simulink model "LevelControl_2025b"  (R2025b)
settings: Solver=FixedStepAuto  StartTime=0.0  StopTime=inf  RelTol=1e-3  EnableMultiTasking=on
libraries: dspstat3 x2, slpidlib x1, arduinolib x1, arduinosensorlib x1
settings Model: ExtModeTrigDuration=2  Creator=Arnt Inge Bøe  LastModifiedBy=Arnt Inge Bøe
settings SolverCC: AutoInsertRateTranBlk=on
settings DataIOCC: ReturnWorkspaceOutputs=off
settings OptimizationCC: EnhancedBackFolding=on  PassReuseOutputArgsAs=Individual arguments  ZeroExternalMemoryAtStartup=off  ZeroInternalMemoryAtStartup=off  MaxStackSize=64  OptimizeBlockOrder=speed  DifferentSizesBufferReuse=on  EfficientTunableParamExpr=on
settings DebuggingCC: ParameterTunabilityLossMsg=error
settings HardwareCC: ProdBitPerPointer=32.0  ProdBitPerSizeT=32.0  ProdBitPerPtrDiffT=32.0  ProdLargestAtomicInteger=Long  ProdLargestAtomicFloat=Double  ProdWordSize=32.0  ProdHWDeviceType=ARM Compatible->ARM Cortex
settings SFSimCC: MATLABDynamicMemAlloc=off
settings RTWCC: SystemTargetFile=ert.tlc  HardwareBoard=Arduino Uno R4 WiFi  TemplateMakefile=ert_default_tmf  Toolchain=Arduino ARM M4  BuildConfiguration=Faster Runs  Description=Embedded Coder
settings CodeAppCC: ForceParamTrailComments=on  IgnoreCustomStorageClasses=off  OperatorAnnotations=on  SimulinkDataObjDesc=on  SFDataObjDesc=on  InsertBlockDesc=on
settings ERTTargetCC: ExtModeTransport=3.0  ExtModeStaticAlloc=on  ExtModeAutomaticAllocSize=off  ExtModeStaticAllocSize=8192.0  ExtModeMexFile=ext_xcp  ExtModeIntrfLevel=Level2 - Open  InlinedParameterPlacement=Hierarchical  SupportContinuousTime=on  SupportVariableSizeSignals=on

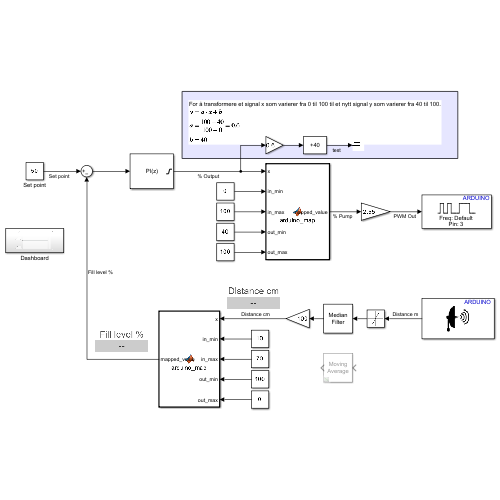
[thumbnail: Simulink's stored preview of the top-level diagram]
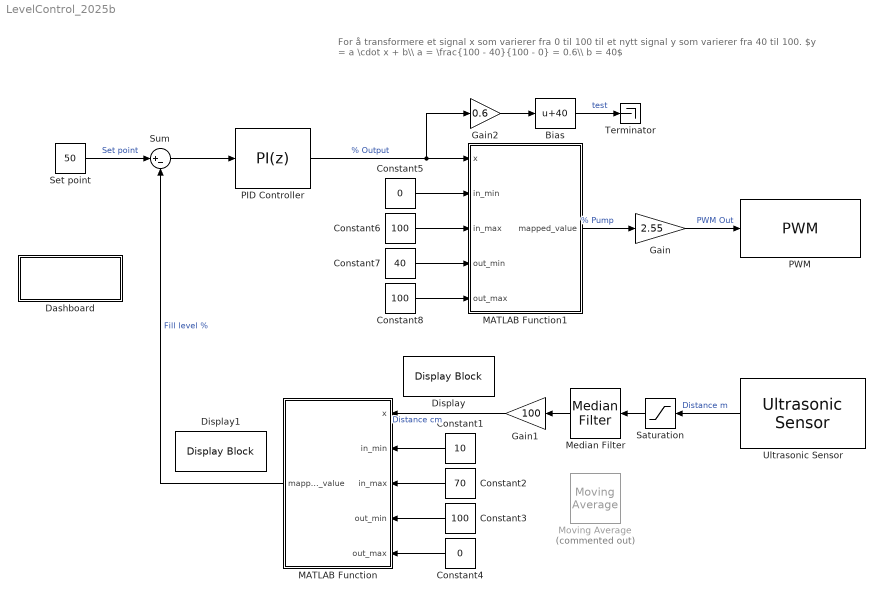
== system LevelControl_2025b ==
  note: For å transformere et signal x som varierer fra 0 til 100 til et nytt signal y som varierer fra 40 til 100.
      | $y = a \cdot x + b\\ a = \frac{100 - 40}{100 - 0} = 0.6\\ b = 40$
  Bias : Bias  Bias=40  SaturateOnIntegerOverflow=off
  Constant1 : Constant  Value=10
  Constant2 : Constant  Value=70
  Constant3 : Constant  Value=100
  Constant4 : Constant  Value=0
  Constant5 : Constant  Value=0
  Constant6 : Constant  Value=100
  Constant7 : Constant  Value=40
  Constant8 : Constant  Value=100
  Dashboard : Subsystem
  Display : DisplayBlock  Transparency=1  FormatString=%d cm  GridColor=[0.502, 0.502, 0.502]
  Display1 : DisplayBlock  Transparency=1  FormatString=%d cm  GridColor=[0.502, 0.502, 0.502]
  Gain : Gain  Gain=2.55  RndMeth=Round
  Gain1 : Gain  Gain=100  RndMeth=Round
  Gain2 : Gain  Gain=0.6
  MATLAB Function : MATLAB Function  TreatAsAtomicUnit=on
  MATLAB Function1 : MATLAB Function  TreatAsAtomicUnit=on
  Median Filter : dspstat3/Median Filter  WindowLength=10  SimulateUsing=Interpreted execution
  Moving Average : dspstat3/Moving Average  Commented=on  Method=Sliding window  ForgettingFactorPort=off  SpecifyWindowLength=on  WindowLength=10  OverlapLength=9  AllowArbitraryInputLength=off  ForgettingFactor=0.9  SimulateUsing=Interpreted execution
  PID Controller : slpidlib/PID Controller  Controller=PI  Form=Parallel  TimeDomain=Discrete-time  UseExternalTs=off  SampleTime=0.1  IntegratorMethod=Forward Euler  FilterMethod=Forward Euler  ControllerParametersSource=internal  P=1  I=0.5  UseKiTs=off  D=0  UseExternalDerivativeSource=off  N=100  UseFilter=on  TunerSelectOption=Transfer Function Based (PID Tuner App)  InitialConditionSource=internal  InitialConditionForIntegrator=0  InitialConditionForFilter=0  DifferentiatorICPrevScaledInput=0  ExternalReset=none  TrackingMode=off  Kt=1  LimitOutput=on  SatLimitsSource=internal  UpperSaturationLimit=100  LowerSaturationLimit=0  LinearizeAsGain=on  AntiWindupMode=clamping  Kb=1  LimitIntegrator=off  UpperIntegratorSaturationLimit=inf  LowerIntegratorSaturationLimit=-inf  RndMeth=Round  POutMin=[]  POutMax=[]  IOutMin=[]  IOutMax=[]  DOutMin=[]  DOutMax=[]  NOutMin=[]  NOutMax=[]  SumOutMin=[]  SumOutMax=[]  SaturationOutMin=[]  SaturationOutMax=[]  PParamMin=[]  PParamMax=[]  IParamMin=[]  IParamMax=[]  DParamMin=[]  DParamMax=[]  NParamMin=[]  NParamMax=[]  KbParamMin=[]  KbParamMax=[]  KtParamMin=[]  KtParamMax=[]  KbOutMin=[]  KbOutMax=[]  KtOutMin=[]  KtOutMax=[]  IntegratorOutMin=[]  IntegratorOutMax=[]  FilterOutMin=[]  FilterOutMax=[]  SumI1OutMin=[]  SumI1OutMax=[]  SumI2OutMin=[]  SumI2OutMax=[]  SumI3OutMin=[]  SumI3OutMax=[]  SumI4OutMin=[]  SumI4OutMax=[]  SumDOutMin=[]  SumDOutMax=[]  DifferentiatorOutMin=[]  DifferentiatorOutMax=[]  FilterDiffOutCoefMin=[]  FilterDiffOutCoefMax=[]  ReciprocalOutMin=[]  ReciprocalOutMax=[]  SumDenOutMin=[]  SumDenOutMax=[]  SumNumOutMin=[]  SumNumOutMax=[]  DivideOutMin=[]  DivideOutMax=[]  UdiffTsProdOutMin=[]  UdiffTsProdOutMax=[]  NTsProdOutMin=[]  NTsProdOutMax=[]  UintegralTsProdOutMin=[]  UintegralTsProdOutMax=[]  UngainTsProdOutMin=[]  UngainTsProdOutMax=[]  ClampingZeroOutDataTypeStr=Inherit: Inherit via back propagation  ClampingZeroOutMin=[]  ClampingZeroOutMax=[]  FilterDenConstantOutDataTypeStr=Inherit: Inherit via back propagation  FilterDenConstantOutMin=[]  FilterDenConstantOutMax=[]  PCopyOutDataTypeStr=Inherit: Inherit via back propagation  PCopyOutMin=[]  PCopyOutMax=[]  NCopyOutDataTypeStr=Inherit: Inherit via back propagation  NCopyOutMin=[]  NCopyOutMax=[]  IntegratorContinuousStateAttributes=''  IntegratorStateMustResolveToSignalObject=off  IntegratorRTWStateStorageClass=Auto  FilterContinuousStateAttributes=''  FilterStateMustResolveToSignalObject=off  FilterRTWStateStorageClass=Auto  ParallelPVariant=InternalParameters  IdealPVariant=Disabled  IVariant=InternalParameters  DVariant=Disabled  IntegratorVariant=Discrete  SatVariant=Enabled  AWVariant=DiscClampingParallel  PCopyVariant=Disabled  TRVariant=Disabled  FdbkBlocksVariant=Forward  IdealPFdbkVariant=Disabled  SatFdbkVariant=Disabled  DerivativeFilterVariant=Disabled  NVariant=Disabled  NCopyVariant=Disabled_SignalSpec  FilterICVariant=Disabled  IntegratorICVariant=InternalICs  ExternalResetVariant=Disabled  TRSumVariant=Passthrough  SumFdbkVariant=Disabled  SumVariant=Sum_PI  TsampFilterVariant=InternalTs  TsampNgainVariant=Passthrough  TsampIntegralVariant=Disabled_SignalSpec  ExternalSaturationOutDataTypeStr=Inherit: Same as second input  DerivativeSourceVariant=Disabled  PreIntVariant=InternalPreInt
  PWM : arduinolib/PWM  pinNumber=3  frequencyType=Default  desiredFrequency=490.2  achievableFrequency=490.2
  Saturation : Saturate  UpperLimit=0.7  LowerLimit=0.1  RndMeth=Round
  Set point : Constant  Value=50
  Sum : Sum  Inputs=|+-
  Terminator : Terminator
  Ultrasonic Sensor : arduinosensorlib/Ultrasonic Sensor  NumSignalPins=2  TrigPin=4  EchoPin=5  SignalPin=3  SampleTime_=0.1  blockPlatform=ARDUINO
  wires:
  Ultrasonic Sensor/1 -> Saturation/1  "Distance m"
  Gain1/1 -> MATLAB Function/1(x)  "Distance cm"
  Set point/1 -> Sum/1  "Set point"
  PID Controller/1 -> Gain2/1, MATLAB Function1/1(x)  "% Output"
  Constant2/1 -> MATLAB Function/3(in_max)
  Constant1/1 -> MATLAB Function/2(in_min)
  Constant3/1 -> MATLAB Function/4(out_min)
  Constant4/1 -> MATLAB Function/5(out_max)
  MATLAB Function/1(mapped_value) -> Sum/2  "Fill level %"
  Median Filter/1 -> Gain1/1
  Constant5/1 -> MATLAB Function1/2(in_min)
  Constant7/1 -> MATLAB Function1/4(out_min)
  Constant8/1 -> MATLAB Function1/5(out_max)
  Constant6/1 -> MATLAB Function1/3(in_max)
  MATLAB Function1/1(mapped_value) -> Gain/1  "% Pump"
  Gain/1 -> PWM/1  "PWM Out"
  Saturation/1 -> Median Filter/1
  Sum/1 -> PID Controller/1
  Gain2/1 -> Bias/1
  Bias/1 -> Terminator/1  "test"

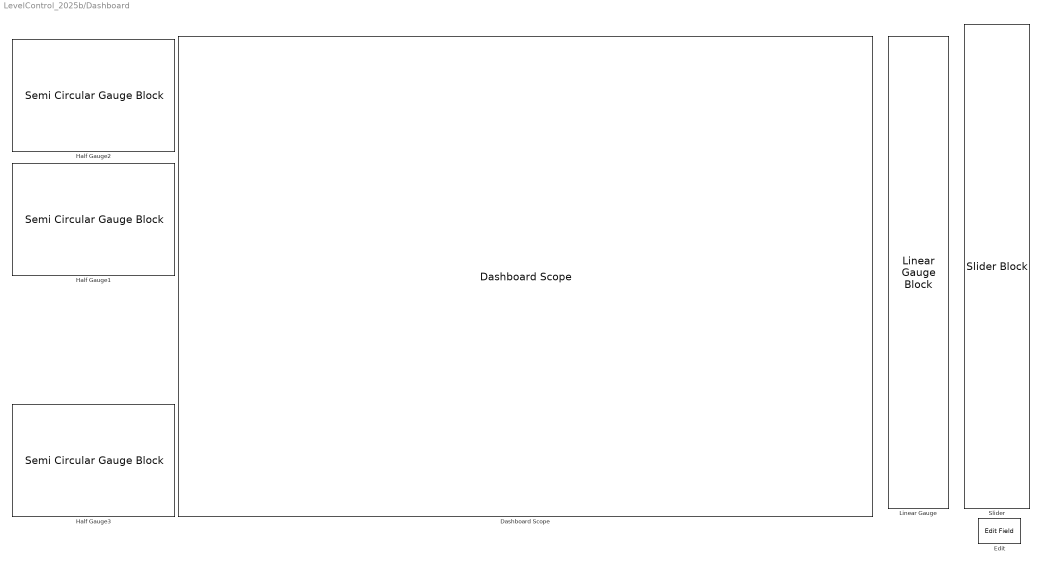
== system LevelControl_2025b/Dashboard ==
  Dashboard Scope : DashboardScope  TimeSpan=60  Ymin=0  Ymax=101  ScaleAtStop=off  UpdateMode=Scroll  FontColor=[0.0, 0.0, 0.0]
  Edit : EditField  LabelPosition=Hide  ShowInitialText=on  Alignment=Center
  Half Gauge1 : SemiCircularGaugeBlock  FontColor=[0.0, 0.0, 0.0]
  Half Gauge2 : SemiCircularGaugeBlock  FontColor=[0.0, 0.0, 0.0]
  Half Gauge3 : SemiCircularGaugeBlock  FontColor=[0.0, 0.0, 0.0]
  Linear Gauge : LinearGaugeBlock  TickInterval=5  FontColor=[0.0, 0.0, 0.0]
  Slider : SliderBlock  TickInterval=5

== matlab function LevelControl_2025b/MATLAB Function1 ==
  data: x input; mapped_value output; in_min input; in_max input; out_min input; out_max input
function mapped_value = arduino_map(x, in_min, in_max, out_min, out_max)
    % Replicates Arduino's map() function
    mapped_value = ((x - in_min) * (out_max - out_min)) / (in_max - in_min) + out_min;
    
    % Clamp the result to [0, 100]
    mapped_value = max(0, min(100, mapped_value));

    % Round to 0.1 decimal places
    mapped_value = round(mapped_value * 10) / 10;
end

== matlab function LevelControl_2025b/MATLAB Function ==
  data: x input; mapped_value output; in_min input; in_max input; out_min input; out_max input
function mapped_value = arduino_map(x, in_min, in_max, out_min, out_max)
    % Replicates Arduino's map() function
    mapped_value = ((x - in_min) * (out_max - out_min)) / (in_max - in_min) + out_min;
    
    % Clamp the result to [0, 100]
    mapped_value = max(0, min(100, mapped_value));

    % Round to 0.1 decimal places
    mapped_value = round(mapped_value * 10) / 10;
end
